simulink model "A2_18"  (R2021a)
settings: Solver=VariableStepAuto  StartTime=0.0  StopTime=100000  RelTol=1e-3
values from neighbouring files (symbols this model uses):
  g = 98.1    [A2_18_data.m]
  K1 = 188/60    (= 3.13333333333)    [A2_18_data.m]
  K2 = 0.012    [A2_18_data.m]
  K3 = 24.9/60    (= 0.415)    [A2_18_data.m]
  r = 2.4    [A2_18_data.m]
settings Model: Creator=Nils Kutter  LastModifiedBy=kbhan

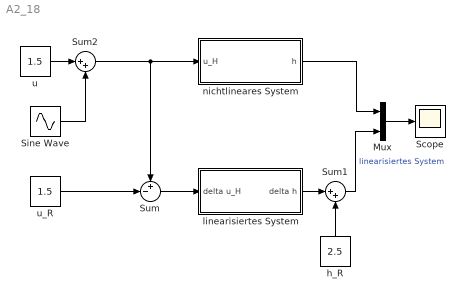
== system A2_18 ==
  Mux : Mux  Inputs=2
  Scope : Scope
  Sine Wave : Sin  Frequency=0.001  SampleTime=0
  Sum : Sum  Inputs=+-|
  Sum1 : Sum  Inputs=|++
  Sum2 : Sum  Inputs=|++
  h_R : Constant  Value=2.5
  linearisiertes System : Subsystem
  nichtlineares System : Subsystem
  u : Constant  Value=1.5
  u_R : Constant  Value=1.5
  wires:
  Sine Wave/1 -> Sum2/2
  linearisiertes System/1(delta h) -> Sum1/1
  u_R/1 -> Sum/2
  Mux/1 -> Scope/1
  Sum1/1 -> Mux/2  "linearisiertes System"
  h_R/1 -> Sum1/2
  nichtlineares System/1(h) -> Mux/1
  u/1 -> Sum2/1
  Sum/1 -> linearisiertes System/1(delta u_H)
  Sum2/1 -> nichtlineares System/1(u_H), Sum/1

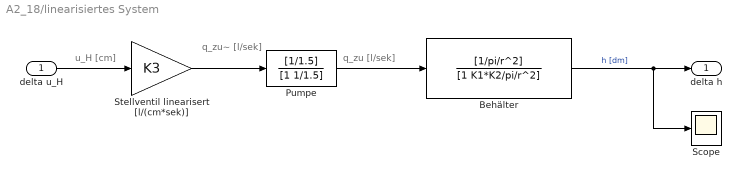
== system A2_18/linearisiertes System ==
  note: u_H [cm]
  note: q_zu~ [l/sek]
  note: q_zu [l/sek]
  delta u_H : Inport
  Behälter : TransferFcn  Numerator=[1/pi/r^2]  Denominator=[1 K1*K2/pi/r^2]
  Pumpe : TransferFcn  Numerator=[1/1.5]  Denominator=[1 1/1.5]
  Scope : Scope
  Stellventil linearisert [l/(cm*sek)] : Gain  Gain=K3
  delta h : Outport
  wires:
  Stellventil linearisert [l/(cm*sek)]/1 -> Pumpe/1
  Pumpe/1 -> Behälter/1
  delta u_H/1 -> Stellventil linearisert [l/(cm*sek)]/1
  Behälter/1 -> Scope/1, delta h/1  "h [dm]"

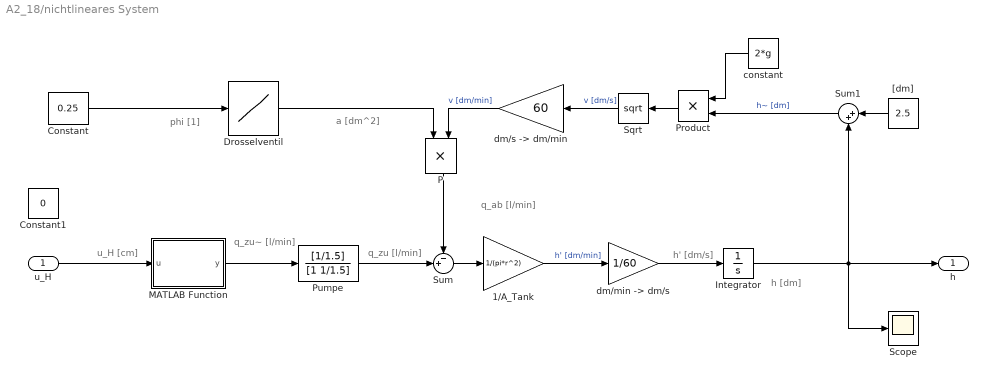
== system A2_18/nichtlineares System ==
  note: u_H [cm]
  note: q_zu~ [l/min]
  note: phi [1]
  note: a [dm^2]
  note: q_zu [l/min]
  note: q_ab [l/min]
  note: h [dm]
  note: h' [dm/s]
  u_H : Inport
  1/A_Tank : Gain  Gain=1/(pi*r^2)
  Constant : Constant  Value=0.25
  Constant1 : Constant  Value=0
  Drosselventil : Lookup  InputValues=[0 0.05 0.1 0.15 0.2 0.25 0.3 0.35 0.4 0.45 0.5]  Table=[0 0.001 0.003 0.005 0.008 0.012 0.017 0.022 0.03 0.039 0.05]
  Integrator : Integrator  InitialCondition=2.5  LowerSaturationLimit=0
  MATLAB Function : MATLAB Function  TreatAsAtomicUnit=on
  P : Product  RndMeth=Zero
  Product : Product
  Pumpe : TransferFcn  Numerator=[1/1.5]  Denominator=[1 1/1.5]
  Scope : Scope
  Sqrt : Sqrt  SaturateOnIntegerOverflow=on
  Sum : Sum  Inputs=-+|
  Sum1 : Sum  Inputs=|++
  "[dm]" : Constant  Value=2.5
  constant : Constant  Value=2*g
  "dm/min -> dm/s" : Gain  Gain=1/60
  "dm/s -> dm/min" : Gain  Gain=60
  h : Outport
  wires:
  P/1 -> Sum/1
  MATLAB Function/1(y) -> Pumpe/1
  Pumpe/1 -> Sum/2
  Sum/1 -> 1/A_Tank/1
  1/A_Tank/1 -> "dm/min -> dm/s"/1  "h' [dm/min]"
  Integrator/1 -> Scope/1, h/1, Sum1/2
  Sum1/1 -> Product/2  "h~ [dm]"
  "[dm]"/1 -> Sum1/1
  Constant/1 -> Drosselventil/1
  Drosselventil/1 -> P/1
  Sqrt/1 -> "dm/s -> dm/min"/1  "v [dm/s]"
  "dm/s -> dm/min"/1 -> P/2  "v [dm/min]"
  "dm/min -> dm/s"/1 -> Integrator/1
  constant/1 -> Product/1
  Product/1 -> Sqrt/1
  u_H/1 -> MATLAB Function/1(u)

== matlab function A2_18/nichtlineares System/MATLAB Function ==
  data: u input; y output
function y = fcn(u)
y = 10*u*(u<0.3)*(u>=0)+(10*u^1.8+1.85)*(u>=0.3);
